simulink model "fuzzy_pid_sim"  (R2020a)
settings: Solver=FixedStepAuto  StartTime=1  StopTime=1  FixedStep=0.0001  RelTol=1e-3
libraries: fuzblock x1
settings Model: Creator=Love Panta  LastModifiedBy=Love Panta

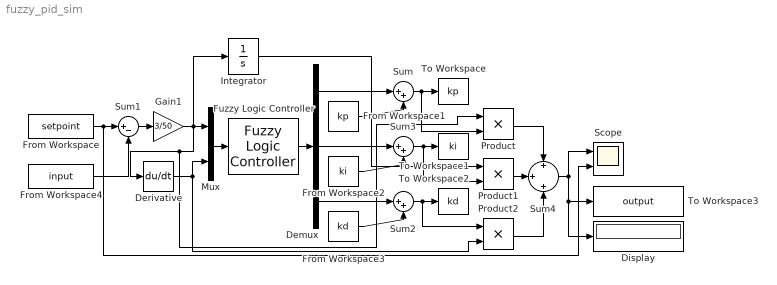
== system fuzzy_pid_sim ==
  Demux : Demux  Outputs=3
  Derivative : Derivative
  Display : Display
  From Workspace : FromWorkspace  VariableName=setpoint
  From Workspace1 : FromWorkspace  VariableName=kp
  From Workspace2 : FromWorkspace  VariableName=ki
  From Workspace3 : FromWorkspace  VariableName=kd
  From Workspace4 : FromWorkspace  VariableName=input
  Fuzzy Logic Controller : fuzblock/Fuzzy Logic  Controller  FIS='fuzzy_test.fis'  OutputSampleNumber=101  DataType=double  FuzzifiedInputs=off  RuleFiringStrengths=off  RuleOutputs=off  AggregatedOutputs=off  SimulateUsing=Interpreted execution  OutOfRangeInputValueMessage=warning  NoRuleFiredMessage=warning  EmptyOutputFuzzySetMessage=warning
  Gain1 : Gain  Gain=3/50
  Integrator : Integrator
  Mux : Mux  Inputs=2
  Product : Product
  Product1 : Product
  Product2 : Product
  Scope : Scope  NumInputPorts=2
  Sum : Sum  Inputs=|++
  Sum1 : Sum  Inputs=|+-
  Sum2 : Sum  Inputs=|++
  Sum3 : Sum  Inputs=|++
  Sum4 : Sum  Inputs=+|+|+
  To Workspace : ToWorkspace  VariableName=kp  SaveFormat=Timeseries  SampleTime=-1
  To Workspace1 : ToWorkspace  VariableName=ki  SaveFormat=Timeseries  SampleTime=-1
  To Workspace2 : ToWorkspace  VariableName=kd  SaveFormat=Timeseries  SampleTime=-1
  To Workspace3 : ToWorkspace  VariableName=output  SaveFormat=Timeseries  SampleTime=-1
  wires:
  From Workspace/1 -> Sum1/1, Scope/2
  Sum1/1 -> Gain1/1
  Fuzzy Logic Controller/1 -> Demux/1
  Demux/1 -> Sum/1
  Demux/2 -> Sum3/1
  Demux/3 -> Sum2/1
  From Workspace1/1 -> Sum/2
  From Workspace2/1 -> Sum3/2
  From Workspace3/1 -> Sum2/2
  Product2/1 -> Sum4/3
  Mux/1 -> Fuzzy Logic Controller/1
  Sum4/1 -> Scope/1, Display/1, To Workspace3/1
  Sum/1 -> To Workspace/1, Product/2
  Sum3/1 -> To Workspace1/1, Product1/2
  Sum2/1 -> To Workspace2/1, Product2/1
  Product1/1 -> Sum4/2
  Product/1 -> Sum4/1
  From Workspace4/1 -> Sum1/2
  Gain1/1 -> Derivative/1, Product/1, Integrator/1, Mux/1
  Integrator/1 -> Product1/1
  Derivative/1 -> Mux/2, Product2/2
